simulink model "simulation_gripen_roo"  (R2021a)
settings: Solver=ode15s  StartTime=0.0  StopTime=200  RelTol=1e-3  EnableMultiTasking=on
values from neighbouring files (symbols this model uses):
  A = [-0.292 -0.152 0.0364 0 0 0 0 8.13 -2.54 -0.0678 1 0 ... (49 elements, 7x7)]    [Gripendata.mat]
  B = [0 -31.7 0 0 0 20 0 -2.15 0.0274 1.48 0 0 ... (14 elements, 7x2)]    [Gripendata.mat]
  C = [0 0 0 0 0 0 1 0 0 1 0 0 ... (14 elements, 2x7)]    [Gripendata.mat]
  D = [0  0; 0  0]    [Gripendata.mat]
  x0 = [5 0.00174532925199 0.00174532925199 0.0872664625997 0.0872664625997 0 0]    [Gripendata.mat]
undefined symbols (not defined in the file or in its folder): A_xi, B_xi, Ken_eta, Ken_x, Lt
settings Model: Creator=scattolini  LastModifiedBy=fabio
settings SolverCC: AlgebraicLoopSolver=TrustRegion
settings DataIOCC: LimitDataPoints=on  SaveFormat=Array  SignalLoggingSaveFormat=ModelDataLogs  ReturnWorkspaceOutputs=off
settings OptimizationCC: ExpressionDepthLimit=2147483647  InitFltsAndDblsToZero=on  LifeSpan=inf
settings DebuggingCC: SaveWithParameterizedLinksMsg=none  UnderspecifiedInitializationDetection=Classic  MergeDetectMultiDrivingBlocksExec=none  SignalResolutionControl=TryResolveAllWithWarning  SolverPrmCheckMsg=warning  MultiTaskDSMMsg=warning  MultiTaskCondExecSysMsg=none  FcnCallInpInsideContextMsg=warning  StateNameClashWarn=warning  SFUnexpectedBacktrackingDiag=warning  SFNoUnconditionalDefaultTransitionDiag=warning  SFExecutionAtInitializationDiag=none  SFMachineParentedDataDiag=warning  ArithmeticOperatorsInVariantConditions=warning
settings HardwareCC: ProdBitPerPointer=32  ProdBitPerSizeT=32  ProdBitPerPtrDiffT=32  ProdLargestAtomicFloat=None  ProdIntDivRoundTo=Undefined  ProdEndianess=Unspecified  ProdWordSize=32  ProdHWDeviceType=32-bit Generic
settings ModelReferenceCC: PropagateSignalLabelsOutOfModel=off
settings SFSimCC: SimUseLocalCustomCode=off  CustomCodeUndefinedFunction=UseInterfaceOnly
settings RTWCC: RTWUseLocalCustomCode=off
settings CodeAppCC: StateflowObjectComments=on
settings GRTTargetCC: TargetFcnLib=ansi_tfl_tmw.mat  TargetLangStandard=C89/C90 (ANSI)  CombineOutputUpdateFcns=off  GRTInterface=on
settings ConfigComp: CovMetricSettings=dw  CovSaveCumulativeToWorkspaceVar=on  CovSaveSingleToWorkspaceVar=on  CovExternalEMLEnable=off

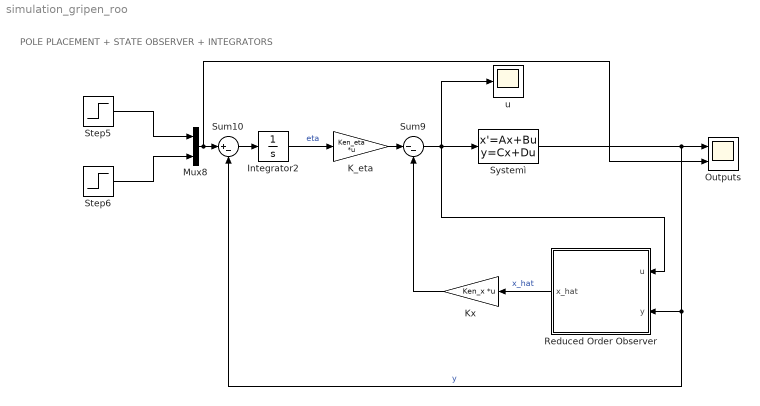
== system simulation_gripen_roo ==
  note: POLE PLACEMENT + STATE OBSERVER + INTEGRATORS
  Integrator2 : Integrator
  K_eta : Gain  Gain=Ken_eta  Multiplication=Matrix(K*u) (u vector)
  Kx : Gain  Gain=Ken_x  Multiplication=Matrix(K*u) (u vector)
  Mux8 : Mux  Inputs=2
  Outputs : Scope  NumInputPorts=2
  Reduced Order Observer : Subsystem
  Step5 : Step  Time=100  After=1.04  SampleTime=0
  Step6 : Step  Time=150  After=-0.52  SampleTime=0
  Sum10 : Sum  Inputs=|+-
  Sum9 : Sum  Inputs=|--
  Systemì : StateSpace  A=A  B=B  C=C  D=D  InitialCondition=x0
  u : Scope
  wires:
  Systemì/1 -> Reduced Order Observer/2(y), Sum10/2, Outputs/1  "y"
  Sum9/1 -> u/1, Reduced Order Observer/1(u), Systemì/1
  Reduced Order Observer/1(x_hat) -> Kx/1  "x_hat"
  Sum10/1 -> Integrator2/1
  Mux8/1 -> Outputs/2, Sum10/1
  K_eta/1 -> Sum9/1
  Step5/1 -> Mux8/1
  Integrator2/1 -> K_eta/1  "eta"
  Step6/1 -> Mux8/2
  Kx/1 -> Sum9/2

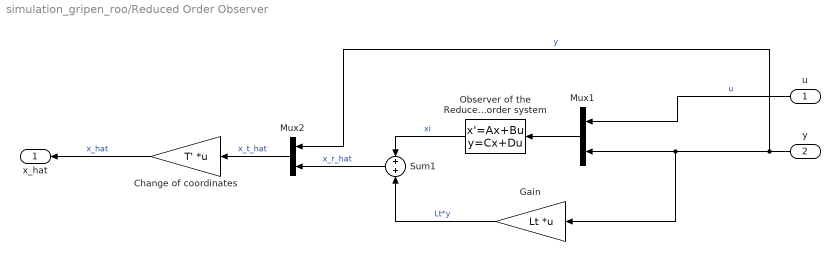
== system simulation_gripen_roo/Reduced Order Observer ==
  u : Inport
  y : Inport  Port=2
  Change of coordinates : Gain  Gain=T'  Multiplication=Matrix(K*u) (u vector)
  Gain : Gain  Gain=Lt  Multiplication=Matrix(K*u) (u vector)
  Mux1 : Mux  Inputs=2
  Mux2 : Mux  Inputs=2
  Observer of the Reduced order system : StateSpace  A=A_xi  B=B_xi  C=eye(5)  D=zeros(5,4)  InitialCondition=0
  Sum1 : Sum
  x_hat : Outport
  wires:
  y/1 -> Mux2/1, Gain/1, Mux1/2  "y"
  Sum1/1 -> Mux2/2  "x_r_hat"
  Observer of the Reduced order system/1 -> Sum1/1  "xi"
  Gain/1 -> Sum1/2  "Lt*y"
  u/1 -> Mux1/1  "u"
  Mux1/1 -> Observer of the Reduced order system/1
  Mux2/1 -> Change of coordinates/1  "x_t_hat"
  Change of coordinates/1 -> x_hat/1  "x_hat"
